simulink model "untitled1"  (R2019b)
settings: Solver=VariableStepAuto  StartTime=0.0  StopTime=10.0  RelTol=1e-3
libraries: neural x1015
(part 1 of 13)
settings Model: Creator=Laura  LastModifiedBy=Laura

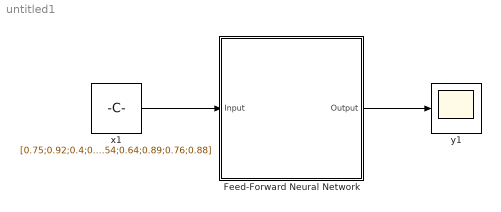
== system untitled1 ==
  Feed-Forward Neural Network : Subsystem
      mask help: Feed-Forward Neural Network
      mask Display: e = 0.06;c1 = [120 150 230]/255;c2 = ([120 150 230]+0)/383;c3 = ([120 150 230]+128)/383;patch([0 1 1 0],[0 0 1 1],c1);patch([0 1 1 1-e 1-e 0+e],[0 0 1 1-e 0+e 0+e],c2);patch([0 0 1 1-e 0+e 0+e],[0 1 1 1-e 1-e 0+e],c3);plot([0 1 1 0 0],[0 0 1 1 0]);fprintf('NNET');port_label('input',1,' Input');port_label('output',1,'Output ');
  x1 : Constant  Value=[0.75;0.92;0.4;0.09;0.94;0.58;0.23;0.34;0.51;0.78;0.15;0.54;0.38;0.16;0.92;0.16;0.4;0.15;0.73;0.99;0.017;0.9;0.34;0.86;0.96;0.56;0.13;0.57;0.49;0.022;0.46;0.53;0.51;0.9;0.15;0.85;0.2;0.35;0.043;0.15;0.23;0.81;0.48;0.5;0.71;0.12;0.54;0.52;0.96;0.18;0.53;0.84;0.67;0.54;0.19;0.13;0.12;0.64;0.17;0.65;0.071;0.95;0.41;0.62;0.18;0.6;0.58;0.031;0.98;0.58;0.63;0.27;0.32;0.48;0.77;0.85;0.93;0.75;0.86;0.51;0.66;0.21;0.24;0.64;0.6;0.9;0.92;0.46;0.47;0.17;0.18;0.83;0.14;0.82;0.68;0.29;0.76;0.66;0.062;0.95;0.97;0.24;0.26;0.62;0.24;0.77;0.14;0.98;0.48;0.44;0.24;0.76;0.69;0.51;0.42;0.067;0.92;0.31;1;0.63;0.32;0.16;0.81;0.88;0.59;0.19;0.24;0.54;0.89;0.61;0.17;0.44;0.83;0.84;0.69;0.86;0.63;0.37;0.28;0.9;0.72;0.21;0.2;0.14;0.4;0.082;0.72;0.64;0.75;0.2;0.26;0.064;0.54;0.53;0.29;0.52;0.83;0.86;0.93;0.86;0.4;0.16;0.94;0.97;0.27;0.95;0.96;0.75;0.78;0.57;0.016;0.43;0.63;0.82;0.2;0.41;0.96;0.066;0.41;0.78;0.55;0.68;0.55;0.86;0.32;0.21;0.4;0.81;0.64;0.38;0.34;0.23;0.74;0.019;0.11;0.26;0.61;0.064;0.067;0.44;1;0.45;0.19;0.11;0.27;0.0061;0.25;0.093;0.78;0.96;0.69;0.11;0.89;0.96;0.4;0.85;0.56;0.12;0.54;0.84;0.55;0.44;0.93;0.99;0.45;0.42;0.6;0.34;0.44;0.071;0.18;0.97;0.55;0.46;0.39;0.61;0.47;0.7;0.68;0.67;0.74;0.18;0.3;0.32;0.85;0.86;0.43;0.98;0.77;0.35;0.34;0.52;0.71;0.77;0.97;0.0017;0.83;0.73;0.91;0.48;0.65;0.37;0.42;0.81;0.14;0.24;0.97;0.29;0.18;0.018;0.76;0.26;0.49;0.96;0.54;0.11;0.69;0.32;0.38;0.22;0.39;0.9;0.92;0.58;0.064;0.23;0.6;0.72;0.91;0.46;0.17;0.34;0.81;0.14;0.75;0.77;0.44;0.093;0.39;0.036;0.93;0.75;0.59;0.64;0.18;0.19;0.52;0.58;0.68;0.34;0.32;0.92;0.36;0.26;0.71;0.62;0.29;0.74;0.72;0.05;0.43;0.86;0.71;0.19;0.99;0.63;0.87;0.15;0.69;0.59;0.15;0.54;0.19;0.74;0.29;0.96;0.81;0.22;0.2;0.94;0.051;0.81;0.012;0.086;0.72;0.98;0.58;0.051;0.65;0.33;0.2;0.11;0.53;0.0056;0.068;0.28;0.98;0.39;0.59;0.59;0.33;0.64;0.16;0.66;0.72;0.26;0.45;0.83;0.52;0.84;0.69;0.2;0.046;0.83;0.095;0.48;0.16;0.32;0.098;0.99;0.89;0.37;0.029;0.33;0.4;0.87;0.51;0.32;0.71;0.44;1;0.22;0.36;0.94;0.61;0.66;0.47;0.44;0.43;0.11;0.54;0.87;0.82;0.46;0.52;0.46;0.19;0.86;0.017;0.34;0.26;0.15;0.95;0.32;0.84;0.66;0.33;0.037;0.51;0.61;0.67;0.087;0.17;0.99;0.57;0.98;0.24;0.6;0.92;0.12;0.39;0.79;0.91;0.18;0.11;0.031;0.32;0.86;0.33;0.48;0.94;0.034;0.63;0.81;0.51;0.97;0.87;0.24;0.34;0.046;0.57;0.58;0.033;0.84;0.66;0.92;0.94;0.022;0.089;0.19;0.9;0.86;0.56;0.24;0.88;0.65;0.3;0.47;0.33;0.36;0.76;0.035;0.9;0.2;0.98;0.077;0.22;0.14;0.39;0.71;0.033;0.65;0.49;0.97;0.93;0.3;0.2;0.22;0.98;0.024;0.39;0.25;0.06;0.28;0.089;0.032;0.93;0.14;0.74;0.67;0.93;0.21;0.53;0.2;0.068;0.82;0.45;0.81;0.44;0.33;0.95;0.97;0.42;0.99;0.38;0.87;0.16;0.35;0.41;0.72;0.56;0.35;0.29;0.48;0.86;0.89;0.53;0.96;0.91;0.37;0.16;0.96;0.6;0.36;0.11;0.96;0.0068;0.65;0.19;0.73;0.41;0.28;0.16;0.37;0.08;0.15;0.82;0.47;0.91;0.18;0.78;0.049;0.26;0.72;0.29;0.41;0.29;0.14;0.95;0.42;0.9;0.78;0.92;0.56;0.78;0.056;0.74;0.29;0.025;0.021;0.28;0.53;0.75;0.15;0.96;0.18;0.4;0.54;0.16;0.93;0.19;0.5;0.18;0.4;0.68;0.063;1;0.3;0.68;0.86;0.19;0.86;0.7;0.0095;0.99;0.27;0.82;0.7;0.81;0.28;0.085;0.022;0.2;0.33;0.43;0.6;0.066;0.84;0.4;0.78;0.048;0.06;0.12;0.2;0.32;0.73;0.55;0.44;0.31;0.024;0.92;0.2;0.66;0.15;0.22;0.2;0.78;0.36;0.65;0.047;0.044;0.038;0.59;0.67;0.97;0.2;0.33;0.55;0.69;0.87;0.12;0.14;0.082;0.55;0.21;0.23;0.56;0.78;0.12;0.22;0.83;0.34;0.27;0.89;0.9;0.87;0.53;0.46;0.55;0.81;0.28;0.13;0.76;0.12;0.77;0.91;0.97;0.56;0.27;0.62;0.47;0.13;0.42;0.69;0.89;0.039;0.99;0.97;0.7;0.66;0.59;0.99;0.82;0.28;0.28;0.87;0.5;0.4;0.59;0.64;0.46;0.46;0.91;0.55;0.56;0.29;0.14;0.32;0.61;0.72;0.89;0.31;0.91;0.55;0.12;0.046;0.043;0.038;0.28;0.95;0.51;0.82;0.79;0.65;0.16;0.41;0.71;0.45;0.25;0.045;0.96;0.73;0.8;0.47;0.79;0.096;0.42;0.084;0.77;0.26;0.62;0.15;0.25;0.58;0.0084;0.046;0.92;0.71;0.41;0.8;0.8;0.85;0.75;0.86;0.33;0.4;0.24;0.47;0.8;0.13;0.79;0.88;0.09;0.075;0.45;0.51;0.87;0.28;0.74;0.97;0.86;0.7;0.23;0.045;0.34;0.91;0.71;0.97;0.018;0.33;0.51;0.49;0.57;0.96;0.94;0.013;0.55;0.19;0.49;0.021;0.67;0.046;0.18;0.35;0.88;0.24;0.9;0.88;0.71;0.15;0.99;0.074;0.23;0.99;0.6;0.29;0.095 ...(+1015 chars)]  SampleTime=0.1
      mask Display: e = 0.06;c1 = [120 230 180]/255;c2 = ([120 230 180]+0)/(256+128);c3 = ([120 230 180]+128)/(256+128);patch([0 1 1 0],[0 0 1 1],c1);patch([0 1 1 1-e 1-e 0+e],[0 0 1 1-e 0+e 0+e],c2);patch([0 0 1 1-e 0+e 0+e],[0 1 1 1-e 1-e 0+e],c3);plot([0 1 1 0 0],[0 0 1 1 0]);disp('Constant');
  y1 : Scope
      mask Display: e = 0.06;c1 = [120 230 180]/255;c2 = ([120 230 180]+0)/(256+128);c3 = ([120 230 180]+128)/(256+128);patch([0 1 1 0],[0 0 1 1],c1);patch([0 1 1 1-e 1-e 0+e],[0 0 1 1-e 0+e 0+e],c2);patch([0 0 1 1-e 0+e 0+e],[0 1 1 1-e 1-e 0+e],c3);plot([0 1 1 0 0],[0 0 1 1 0]);plot([0.15 0.85 0.85 0.15 0.15],[0.5 0.5 0.85 0.85 0.5]);
  wires:
  x1/1 -> Feed-Forward Neural Network/1(Input)
  Feed-Forward Neural Network/1(Output) -> y1/1

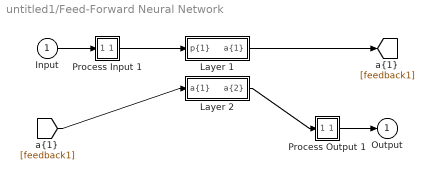
== system untitled1/Feed-Forward Neural Network ==
  Input : Inport  PortDimensions=1001  SampleTime=0.1
      mask Display: e = 0.06;c1 = [120 230 180]/255;c2 = ([120 230 180]+0)/(256+128);c3 = ([120 230 180]+128)/(256+128);patch([0 1 1 0],[0 0 1 1],c1);patch([0 1 1 1-e 1-e 0+e],[0 0 1 1-e 0+e 0+e],c2);patch([0 0 1 1-e 0+e 0+e],[0 1 1 1-e 1-e 0+e],c3);plot([0 1 1 0 0],[0 0 1 1 0]);
  Layer 1 : Subsystem
      mask Display: e = 0.06;c1 = [120 150 230]/255;c2 = ([120 150 230]+0)/383;c3 = ([120 150 230]+128)/383;patch([0 1 1 0],[0 0 1 1],c1);patch([0 1 1 1-e 1-e 0+e],[0 0 1 1-e 0+e 0+e],c2);patch([0 0 1 1-e 0+e 0+e],[0 1 1 1-e 1-e 0+e],c3);plot([0 1 1 0 0],[0 0 1 1 0]);
  Layer 2 : Subsystem
      mask Display: e = 0.06;c1 = [120 150 230]/255;c2 = ([120 150 230]+0)/383;c3 = ([120 150 230]+128)/383;patch([0 1 1 0],[0 0 1 1],c1);patch([0 1 1 1-e 1-e 0+e],[0 0 1 1-e 0+e 0+e],c2);patch([0 0 1 1-e 0+e 0+e],[0 1 1 1-e 1-e 0+e],c3);plot([0 1 1 0 0],[0 0 1 1 0]);
  Process Input 1 : Subsystem
      mask Display: e = 0.06;c1 = [120 150 230]/255;c2 = ([120 150 230]+0)/383;c3 = ([120 150 230]+128)/383;patch([0 1 1 0],[0 0 1 1],c1);patch([0 1 1 1-e 1-e 0+e],[0 0 1 1-e 0+e 0+e],c2);patch([0 0 1 1-e 0+e 0+e],[0 1 1 1-e 1-e 0+e],c3);plot([0 1 1 0 0],[0 0 1 1 0]);
  Process Output 1 : Subsystem
      mask Display: e = 0.06;c1 = [120 150 230]/255;c2 = ([120 150 230]+0)/383;c3 = ([120 150 230]+128)/383;patch([0 1 1 0],[0 0 1 1],c1);patch([0 1 1 1-e 1-e 0+e],[0 0 1 1-e 0+e 0+e],c2);patch([0 0 1 1-e 0+e 0+e],[0 1 1 1-e 1-e 0+e],c3);plot([0 1 1 0 0],[0 0 1 1 0]);
  Output : Outport  InitialOutput=[0;0;0;0;0;0;0;0;0;0;0;0;0;0;0;0;0;0;0;0;0;0;0;0;0;0;0;0;0;0;0;0;0;0;0;0;0;0;0;0;0;0;0;0;0;0;0;0;0;0;0;0;0;0;0;0;0;0;0;0;0;0;0;0;0;0;0;0;0;0;0;0;0;0;0;0;0;0;0;0;0;0;0;0;0;0;0;0;0;0;0;0;0;0;0;0;0;0;0;0;0;0;0;0;0;0;0;0;0;0;0;0;0;0;0;0;0;0;0;0;0;0;0;0;0;0;0;0;0;0;0;0;0;0;0;0;0;0;0;0;0;0;0;0;0;0;0;0;0;0;0;0;0;0;0;0;0;0;0;0;0;0;0;0;0;0;0;0;0;0;0;0;0;0;0;0;0;0;0;0;0;0;0;0;0;0;0;0;0;0;0;0;0;0;0;0;0;0;0;0;0;0;0;0;0;0;0;0;0;0;0;0;0;0;0;0;0;0;0;0;0;0;0;0;0;0;0;0;0;0;0;0;0;0;0;0;0;0;0;0;0;0;0;0;0;0;0;0;0;0;0;0;0;0;0;0;0;0;0;0;0;0;0;0;0;0;0;0;0;0;0;0;0;0;0;0;0;0;0;0;0;0;0;0;0;0;0;0;0;0;0;0;0;0;0;0;0;0;0;0;0;0;0;0;0;0;0;0;0;0;0;0;0;0;0;0;0;0;0;0;0;0;0;0;0;0;0;0;0;0;0;0;0;0;0;0;0;0;0;0;0;0;0;0;0;0;0;0;0;0;0;0;0;0;0;0;0;0;0;0;0;0;0;0;0;0;0;0;0;0;0;0;0;0;0;0;0;0;0;0;0;0;0;0;0;0;0;0;0;0;0;0;0;0;0;0;0;0;0;0;0;0;0;0;0;0;0;0;0;0;0;0;0;0;0;0;0;0;0;0;0;0;0;0;0;0;0;0;0;0;0;0;0;0;0;0;0;0;0;0;0;0;0;0;0;0;0;0;0;0;0;0;0;0;0;0;0;0;0;0;0;0;0;0;0;0;0;0;0;0;0;0;0;0;0;0;0;0;0;0;0;0;0;0;0;0;0;0;0;0;0;0;0;0;0;0;0;0;0;0;0;0;0;0;0;0;0;0;0;0;0;0;0;0;0;0;0;0;0;0;0;0;0;0;0;0;0;0;0;0;0;0;0;0;0;0;0;0;0;0;0;0;0;0;0;0;0;0;0;0;0;0;0;0;0;0;0;0;0;0;0;0;0;0;0;0;0;0;0;0;0;0;0;0;0;0;0;0;0;0;0;0;0;0;0;0;0;0;0;0;0;0;0;0;0;0;0;0;0;0;0;0;0;0;0;0;0;0;0;0;0;0;0;0;0;0;0;0;0;0;0;0;0;0;0;0;0;0;0;0;0;0;0;0;0;0;0;0;0;0;0;0;0;0;0;0;0;0;0;0;0;0;0;0;0;0;0;0;0;0;0;0;0;0;0;0;0;0;0;0;0;0;0;0;0;0;0;0;0;0;0;0;0;0;0;0;0;0;0;0;0;0;0;0;0;0;0;0;0;0;0;0;0;0;0;0;0;0;0;0;0;0;0;0;0;0;0;0;0;0;0;0;0;0;0;0;0;0;0;0;0;0;0;0;0;0;0;0;0;0;0;0;0;0;0;0;0;0;0;0;0;0;0;0;0;0;0;0;0;0;0;0;0;0;0;0;0;0;0;0;0;0;0;0;0;0;0;0;0;0;0;0;0;0;0;0;0;0;0;0;0;0;0;0;0;0;0;0;0;0;0;0;0;0;0;0;0;0;0;0;0;0;0;0;0;0;0;0;0;0;0;0;0;0;0;0;0;0;0;0;0;0;0;0;0;0;0;0;0;0;0;0;0;0;0;0;0;0;0;0;0;0;0;0;0;0;0;0;0;0;0;0;0;0;0;0;0;0;0;0;0;0;0;0;0;0;0;0;0;0;0;0;0;0;0;0;0;0;0;0;0;0;0;0;0;0;0;0;0;0;0;0;0;0;0;0;0;0;0;0;0;0;0;0;0;0;0;0;0;0;0;0;0;0;0;0;0;0;0;0;0;0;0;0;0;0;0;0;0;0;0;0;0;0;0;0;0;0;0;0;0;0;0;0;0;0;0;0;0;0;0;0;0;0;0;0;0;0;0;0;0;0;0;0;0;0;0;0;0;0;0;0;0;0;0;0;0;0;0;0;0;0;0;0;0;0;0;0;0;0;0]
      mask Display: e = 0.06;c1 = [120 230 180]/255;c2 = ([120 230 180]+0)/(256+128);c3 = ([120 230 180]+128)/(256+128);patch([0 1 1 0],[0 0 1 1],c1);patch([0 1 1 1-e 1-e 0+e],[0 0 1 1-e 0+e 0+e],c2);patch([0 0 1 1-e 0+e 0+e],[0 1 1 1-e 1-e 0+e],c3);plot([0 1 1 0 0],[0 0 1 1 0]);
  wires:
  Input/1 -> Process Input 1/1(x)
  Process Output 1/1(y) -> Output/1
  Process Input 1/1(p) -> Layer 1/1("p{1}")
  Layer 1/1("a{1}") -> [feedback1]
  [feedback1] -> Layer 2/1("a{1} ")
  Layer 2/1("a{2}") -> Process Output 1/1(a)

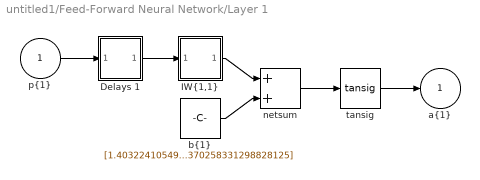
== system untitled1/Feed-Forward Neural Network/Layer 1 ==
  "p{1}" : Inport  PortDimensions=1001  SampleTime=0.1
      mask Display: e = 0.06;c1 = [120 230 180]/255;c2 = ([120 230 180]+0)/(256+128);c3 = ([120 230 180]+128)/(256+128);patch([0 1 1 0],[0 0 1 1],c1);patch([0 1 1 1-e 1-e 0+e],[0 0 1 1-e 0+e 0+e],c2);patch([0 0 1 1-e 0+e 0+e],[0 1 1 1-e 1-e 0+e],c3);plot([0 1 1 0 0],[0 0 1 1 0]);
  Delays 1 : Subsystem
      mask Display: e = 0.06;c1 = [120 150 230]/255;c2 = ([120 150 230]+0)/383;c3 = ([120 150 230]+128)/383;patch([0 1 1 0],[0 0 1 1],c1);patch([0 1 1 1-e 1-e 0+e],[0 0 1 1-e 0+e 0+e],c2);patch([0 0 1 1-e 0+e 0+e],[0 1 1 1-e 1-e 0+e],c3);plot([0 1 1 0 0],[0 0 1 1 0]);disp('0');
  "IW{1,1}" : Subsystem
      mask Display: e = 0.06;c1 = [120 150 230]/255;c2 = ([120 150 230]+0)/383;c3 = ([120 150 230]+128)/383;patch([0 1 1 0],[0 0 1 1],c1);patch([0 1 1 1-e 1-e 0+e],[0 0 1 1-e 0+e 0+e],c2);patch([0 0 1 1-e 0+e 0+e],[0 1 1 1-e 1-e 0+e],c3);plot([0 1 1 0 0],[0 0 1 1 0]);disp('W');
  "b{1}" : Constant  Value=[1.4032241054902545585036932607181370258331298828125;1.0913965264924201381546708944370038807392120361328125;-0.7795689474945859398502534531871788203716278076171875;-0.4677413684967515195012310869060456752777099609375;-0.155913789498917154663359951882739551365375518798828125;0.155913789498917154663359951882739551365375518798828125;0.4677413684967515195012310869060456752777099609375;-0.7795689474945859398502534531871788203716278076171875;1.0913965264924201381546708944370038807392120361328125;-1.4032241054902545585036932607181370258331298828125]
      mask Display: e = 0.06;c1 = [120 150 230]/255;c2 = ([120 150 230]+0)/383;c3 = ([120 150 230]+128)/383;patch([0 1 1 0],[0 0 1 1],c1);patch([0 1 1 1-e 1-e 0+e],[0 0 1 1-e 0+e 0+e],c2);patch([0 0 1 1-e 0+e 0+e],[0 1 1 1-e 1-e 0+e],c3);plot([0 1 1 0 0],[0 0 1 1 0]);disp('b');
  netsum : Sum  Inputs=2  SaturateOnIntegerOverflow=on  InputSameDT=on  OutDataTypeStr=Inherit: Same as first input
      mask Display: e = 0.06;c1 = [120 150 230]/255;c2 = ([120 150 230]+0)/383;c3 = ([120 150 230]+128)/383;patch([0 1 1 0],[0 0 1 1],c1);patch([0 1 1 1-e 1-e 0+e],[0 0 1 1-e 0+e 0+e],c2);patch([0 0 1 1-e 0+e 0+e],[0 1 1 1-e 1-e 0+e],c3);plot([0 1 1 0 0],[0 0 1 1 0]);disp('+');
  tansig : neural/Transfer Functions/tansig
      settings: SourceProductName=Deep Learning Toolbox
  "a{1}" : Outport  InitialOutput=[0;0;0;0;0;0;0;0;0;0]
      mask Display: e = 0.06;c1 = [120 230 180]/255;c2 = ([120 230 180]+0)/(256+128);c3 = ([120 230 180]+128)/(256+128);patch([0 1 1 0],[0 0 1 1],c1);patch([0 1 1 1-e 1-e 0+e],[0 0 1 1-e 0+e 0+e],c2);patch([0 0 1 1-e 0+e 0+e],[0 1 1 1-e 1-e 0+e],c3);plot([0 1 1 0 0],[0 0 1 1 0]);
  wires:
  "p{1}"/1 -> Delays 1/1("p{1}")
  Delays 1/1("pd{1,1}") -> "IW{1,1}"/1("pd{1,1}")
  "IW{1,1}"/1("iz{1,1}") -> netsum/1
  "b{1}"/1 -> netsum/2
  netsum/1 -> tansig/1
  tansig/1 -> "a{1}"/1
